simulink library "Dampers_Axle1_Independent"  (R2026a)
settings: Solver=VariableStepAuto
libraries: Damper_Basics x2, fl_lib x2
Description:
  | Component of Simscape Vehicle Templates Library
  | 
  | Copyright 2018-2026 The MathWorks, Inc.
settings Model: Creator=smiller  LastModifiedBy=smiller

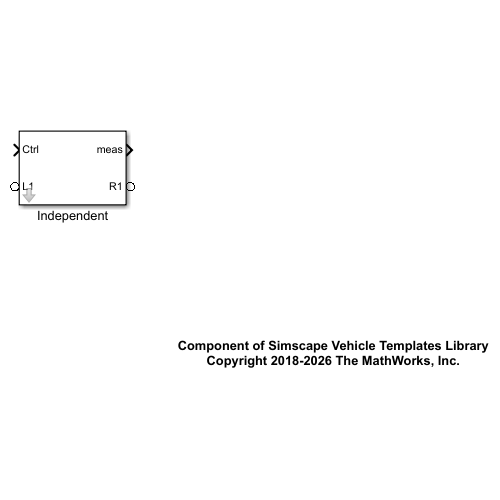
[thumbnail: Simulink's stored preview of the top-level diagram]
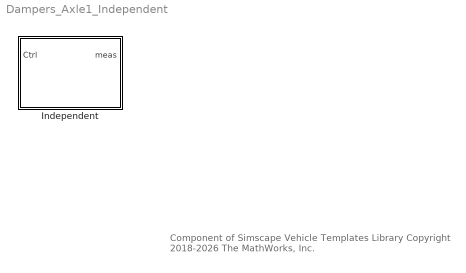
== system Dampers_Axle1_Independent ==
  note: Component of Simscape Vehicle Templates Library
      | Copyright 2018-2026 The MathWorks, Inc.
  Independent : Subsystem  VariantControl=Independent  mask(Independent Dampers){InitTriggerDropdown=0}
      mask prompts: InitTriggerDropdown "Initialization Trigger Dropdown"
      mask help: Models independent left and right dampers.
      mask init:
      | curblk = gcb;
      | 
      | % Trigger Mask Initialization for 
      | % variant subsystems below this level
      | sm_car_lib_maskInitTrigger(curblk);
      mask TypeOptions InitTriggerDropdown: 0 | 1

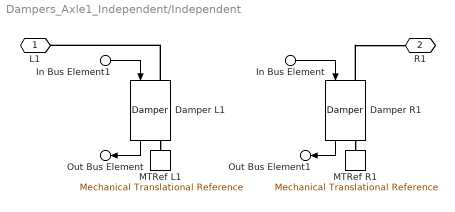
== system Dampers_Axle1_Independent/Independent ==
  In Bus Element1 : Inport  PortName=Ctrl  Element=L1
  In Bus Element : Inport  PortName=Ctrl  Element=R1
  Damper L1 : Damper_Basics/Damper  VariantControl=Variant1  LabelModeActiveChoice=Linear  Damper=Damper.Axle1  VariantLabel=Damper.Axle1.class.Value  InitTriggerDropdown=0
      settings: AttributesFormatString=%<ActiveVariant>
  Damper R1 : Damper_Basics/Damper  VariantControl=Variant1  LabelModeActiveChoice=Linear  Damper=Damper.Axle1  VariantLabel=Damper.Axle1.class.Value  InitTriggerDropdown=0
      settings: AttributesFormatString=%<ActiveVariant>
  MTRef L1 : fl_lib/Mechanical/Translational Elements/Mechanical Translational Reference
  MTRef R1 : fl_lib/Mechanical/Translational Elements/Mechanical Translational Reference
  L1 : PMIOPort  Side=Left
  R1 : PMIOPort  Port=2  Side=Right
  Out Bus Element : Outport  VectorParamsAs1DForOutWhenUnconnected=off  PortName=meas  Element=L1
  Out Bus Element1 : Outport  VectorParamsAs1DForOutWhenUnconnected=off  PortName=meas  Element=R1
  wires:
  In Bus Element/1 -> Damper R1/1
  In Bus Element1/1 -> Damper L1/1
  Damper L1/1 -> Out Bus Element/1
  Damper R1/1 -> Out Bus Element1/1
  connections:
  Damper R1/LConn1 -- R1/RConn1
  Damper R1/RConn1 -- MTRef R1/LConn1
  Damper L1/LConn1 -- L1/RConn1
  Damper L1/RConn1 -- MTRef L1/LConn1
